simulink model "q_2dof_helicopter_quick_start"  (Simulink 8.7)
settings: Solver=ode1  StartTime=0.0  StopTime=inf  FixedStep=0.002  MaxStep=10  RelTol=1e-3  AbsTol=1e-3
libraries: sldrtlib x4, simulink_extras x4, simulink x1
settings Model: Creator=MLevis  LastModifiedBy=lukas  SimulationMode=external  ExtModeTrigDuration=50000
settings SolverCC: PositivePriorityOrder=on
settings DataIOCC: LimitDataPoints=off  SignalLoggingSaveFormat=ModelDataLogs  SaveOutput=off  SaveTime=off  SignalLoggingName=sigsOut
settings OptimizationCC: BlockReduction=off  BooleanDataType=off  OptimizeBlockIOStorage=off  BufferReuse=off  GlobalBufferReuse=off  ExpressionFolding=off  ExpressionDepthLimit=2147483647  LocalBlockOutputs=off  InitFltsAndDblsToZero=on
settings DebuggingCC: SaveWithParameterizedLinksMsg=none  SignalResolutionControl=TryResolveAllWithWarning  MultiTaskDSMMsg=warning  MultiTaskCondExecSysMsg=none  FcnCallInpInsideContextMsg=UseLocalSettings  StateNameClashWarn=warning  StrictBusMsg=None
settings RTWCC: SystemTargetFile=quarc_windows.tlc  TemplateMakefile=quarc_default_tmf  Description=QuaRC Win32 Target
settings STFCustomTargetCC: TargetFcnLib=ansi_tfl_tmw.mat  TargetPreCompLibLocation=C:\PROGRA~2\QUARC\lib\2011a\windows\release  GeneratePreprocessorConditionals=Disable all  CPPClassGenCompliant=on  SystemTargetFile=quarc_windows.tlc
settings GRTTargetCC: TargetFcnLib=ansi_tfl_tmw.mat  TargetPreCompLibLocation=C:\PROGRA~2\QUARC\lib\2011a\windows\release  ParMdlRefBuildCompliant=off  CompOptLevelCompliant=off  ConcurrentExecutionCompliant=off  CombineOutputUpdateFcns=off  MatFileLogging=off  GRTInterface=on  UseToolchainInfoCompliant=off  ExtMode=on  ExtModeMexFile=quarc_comm

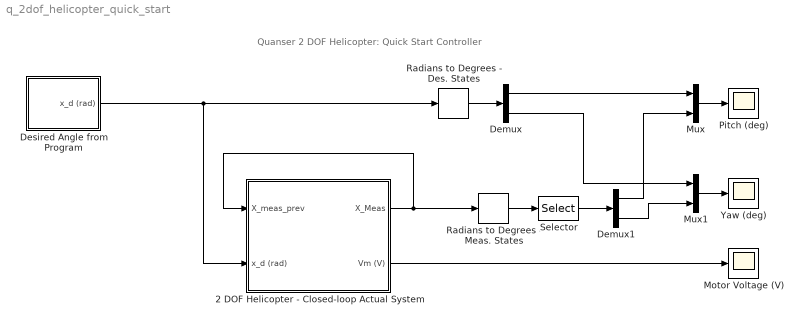
== system q_2dof_helicopter_quick_start ==
  note: Quanser 2 DOF Helicopter:
      | Quick Start Controller
  2 DOF Helicopter - Closed-loop Actual System : Subsystem
  Demux : Demux  Outputs=2
  Demux1 : Demux  Outputs=2
  Desired Angle from Program : Subsystem
  Motor Voltage (V) : Scope
  Mux : Mux  Inputs=2
  Mux1 : Mux  Inputs=2
  Pitch (deg) : Scope
  Radians to Degrees - Des. States : simulink_extras/Transformations/Radians to Degrees
  Radians to Degrees - Meas. States : simulink_extras/Transformations/Radians to Degrees
  Selector : Selector  InputPortWidth=4  IndexOptions=Index vector (dialog)  Indices=[1 2]  OutputSizes=1
  Yaw (deg) : Scope
  wires:
  2 DOF Helicopter - Closed-loop Actual System/1(X_Meas) -> 2 DOF Helicopter - Closed-loop Actual System/1(X_meas_prev), Radians to Degrees - Meas. States/1
  Desired Angle from Program/1(x_d (rad)) -> 2 DOF Helicopter - Closed-loop Actual System/2(x_d (rad)), Radians to Degrees - Des. States/1
  Radians to Degrees - Des. States/1 -> Demux/1
  Radians to Degrees - Meas. States/1 -> Selector/1
  Selector/1 -> Demux1/1
  Mux1/1 -> Yaw (deg)/1
  Mux/1 -> Pitch (deg)/1
  Demux/1 -> Mux/1
  Demux/2 -> Mux1/1
  Demux1/1 -> Mux/2
  Demux1/2 -> Mux1/2
  2 DOF Helicopter - Closed-loop Actual System/2(Vm (V)) -> Motor Voltage (V)/1

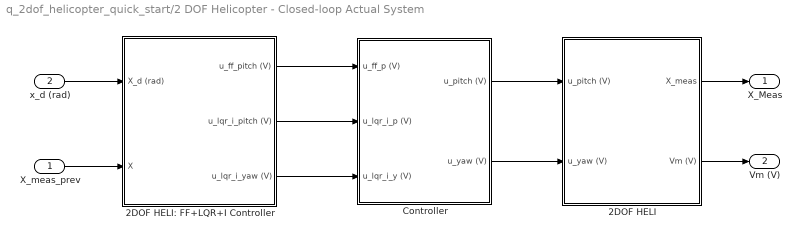
== system q_2dof_helicopter_quick_start/2 DOF Helicopter - Closed-loop Actual System ==
  X_meas_prev : Inport
  x_d (rad) : Inport  Port=2
  2DOF HELI : Subsystem
  2DOF HELI: FF+LQR+I Controller : Subsystem
  "Controller " : Subsystem
  X_Meas : Outport
  Vm (V) : Outport  Port=2
  wires:
  2DOF HELI/1(X_meas) -> X_Meas/1
  x_d (rad)/1 -> 2DOF HELI: FF+LQR+I Controller/1(X_d (rad))
  X_meas_prev/1 -> 2DOF HELI: FF+LQR+I Controller/2(X)
  "Controller "/1(u_pitch (V)) -> 2DOF HELI/1(u_pitch (V))
  "Controller "/2(u_yaw (V)) -> 2DOF HELI/2(u_yaw (V))
  2DOF HELI: FF+LQR+I Controller/2(u_lqr_i_pitch (V)) -> "Controller "/2(u_lqr_i_p (V))
  2DOF HELI: FF+LQR+I Controller/1(u_ff_pitch (V)) -> "Controller "/1(u_ff_p (V))
  2DOF HELI: FF+LQR+I Controller/3(u_lqr_i_yaw (V)) -> "Controller "/3(u_lqr_i_y (V))
  2DOF HELI/2(Vm (V)) -> Vm (V)/1

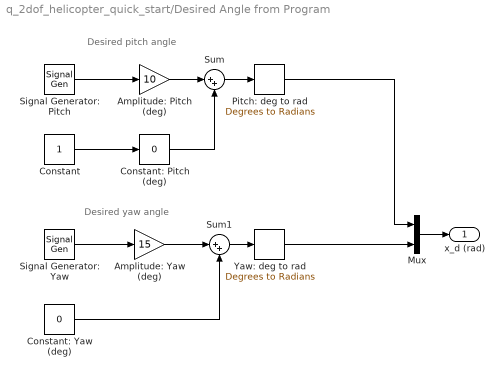
== system q_2dof_helicopter_quick_start/Desired Angle from Program ==
  note: Desired pitch angle
  note: Desired yaw angle
  Amplitude: Pitch (deg) : Gain  Gain=10
  Amplitude: Yaw (deg) : Gain  Gain=15
  Constant : Constant
  Constant: Pitch (deg) : simulink/Math Operations/Slider Gain  low=-30  gain=0  high=15
  Constant: Yaw (deg) : Constant  Value=0
  Mux : Mux  Inputs=2
  Pitch: deg to rad : simulink_extras/Transformations/Degrees to Radians
  Signal Generator: Pitch : SignalGenerator  WaveForm=square  Frequency=0.05
  Signal Generator: Yaw : SignalGenerator  WaveForm=square  Frequency=0.05
  Sum : Sum  Inputs=|++
  Sum1 : Sum  Inputs=|++
  Yaw: deg to rad : simulink_extras/Transformations/Degrees to Radians
  x_d (rad) : Outport
  wires:
  Pitch: deg to rad/1 -> Mux/1
  Sum/1 -> Pitch: deg to rad/1
  Signal Generator: Pitch/1 -> Amplitude: Pitch (deg)/1
  Amplitude: Pitch (deg)/1 -> Sum/1
  Constant/1 -> Constant: Pitch (deg)/1
  Sum1/1 -> Yaw: deg to rad/1
  Signal Generator: Yaw/1 -> Amplitude: Yaw (deg)/1
  Amplitude: Yaw (deg)/1 -> Sum1/1
  Constant: Yaw (deg)/1 -> Sum1/2
  Mux/1 -> x_d (rad)/1
  Yaw: deg to rad/1 -> Mux/2
  Constant: Pitch (deg)/1 -> Sum/2

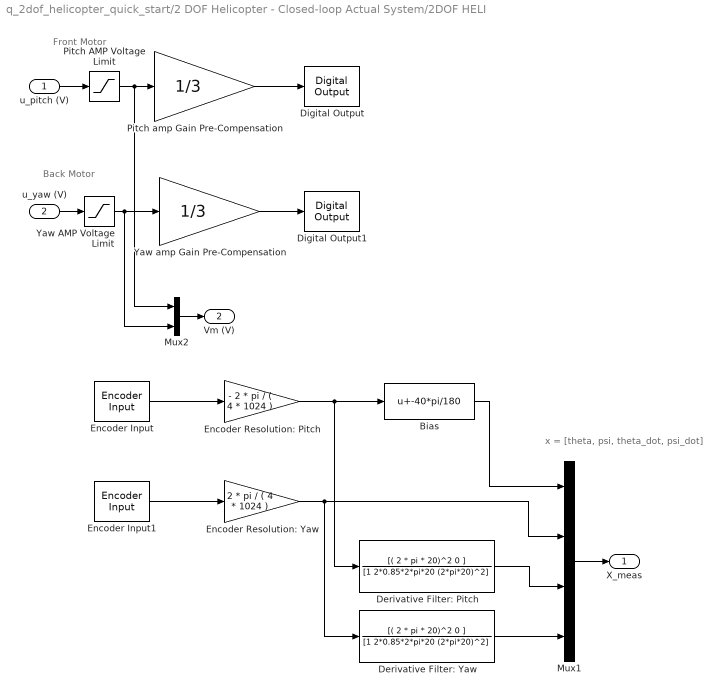
== system q_2dof_helicopter_quick_start/2 DOF Helicopter - Closed-loop Actual System/2DOF HELI ==
  note: Back Motor
  note: Front Motor
  note: x = [theta, psi, theta_dot, psi_dot]
  u_pitch (V) : Inport
  u_yaw (V) : Inport  Port=2
  Bias : Bias  Bias=-40*pi/180
  Derivative Filter: Pitch : TransferFcn  Numerator=[( 2 * pi * 20)^2 0 ]  Denominator=[1 2*0.85*2*pi*20 (2*pi*20)^2]
  Derivative Filter: Yaw : TransferFcn  Numerator=[( 2 * pi * 20)^2 0 ]  Denominator=[1 2*0.85*2*pi*20 (2*pi*20)^2]
  Digital Output : sldrtlib/Digital Output  SampleTime=0.1  MaxMissedTicks=10  ShowMissedTicks=off  YieldWhenWaiting=off  DrvAddress=0  DrvOptions=0  Channels=1  BitMode=1  InitialValue=[]  FinalValue=[]
  Digital Output1 : sldrtlib/Digital Output  SampleTime=0.1  MaxMissedTicks=10  ShowMissedTicks=off  YieldWhenWaiting=off  DrvAddress=0  DrvOptions=0  Channels=1  BitMode=1  InitialValue=[]  FinalValue=[]
  Encoder Input : sldrtlib/Encoder Input  SampleTime=0.01  MaxMissedTicks=10  ShowMissedTicks=off  YieldWhenWaiting=off  DrvAddress=0  DrvOptions=0  Channels=1  QuadMode=3  IndexPulse=2  InputFilter=Inf  DataType=1
  Encoder Input1 : sldrtlib/Encoder Input  SampleTime=0.01  MaxMissedTicks=10  ShowMissedTicks=off  YieldWhenWaiting=off  DrvAddress=0  DrvOptions=0  Channels=1  QuadMode=3  IndexPulse=2  InputFilter=Inf  DataType=1
  "Encoder Resolution: Pitch " : Gain  Gain=- 2 * pi / ( 4 * 1024 )
  Encoder Resolution: Yaw : Gain  Gain=2 * pi / ( 4 * 1024 )
  Mux1 : Mux
  Mux2 : Mux  Inputs=2
  Pitch AMP Voltage Limit : Saturate  UpperLimit=3.5  LowerLimit=-3.5
  Pitch amp Gain Pre-Compensation : Gain  Gain=1/3  SaturateOnIntegerOverflow=on  OutDataTypeStr=Inherit: Same as input  ParamDataTypeStr=Inherit: Same as input
  Yaw AMP Voltage Limit : Saturate  UpperLimit=3.5  LowerLimit=-3.5
  Yaw amp Gain Pre-Compensation : Gain  Gain=1/3  SaturateOnIntegerOverflow=on  OutDataTypeStr=Inherit: Same as input  ParamDataTypeStr=Inherit: Same as input
  X_meas : Outport
  Vm (V) : Outport  Port=2
  wires:
  Encoder Resolution: Yaw/1 -> Mux1/2, Derivative Filter: Yaw/1
  Mux2/1 -> Vm (V)/1
  Yaw amp Gain Pre-Compensation/1 -> Digital Output1/1
  Pitch amp Gain Pre-Compensation/1 -> Digital Output/1
  Mux1/1 -> X_meas/1
  u_yaw (V)/1 -> Yaw AMP Voltage Limit/1
  u_pitch (V)/1 -> Pitch AMP Voltage Limit/1
  Yaw AMP Voltage Limit/1 -> Mux2/2, Yaw amp Gain Pre-Compensation/1
  Pitch AMP Voltage Limit/1 -> Mux2/1, Pitch amp Gain Pre-Compensation/1
  Encoder Input/1 -> "Encoder Resolution: Pitch "/1
  "Encoder Resolution: Pitch "/1 -> Bias/1, Derivative Filter: Pitch/1
  Encoder Input1/1 -> Encoder Resolution: Yaw/1
  Bias/1 -> Mux1/1
  Derivative Filter: Pitch/1 -> Mux1/3
  Derivative Filter: Yaw/1 -> Mux1/4

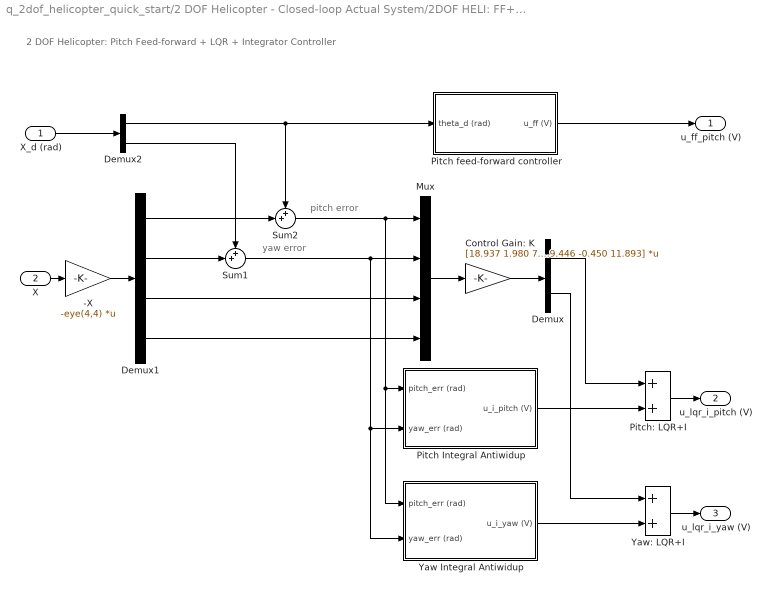
== system q_2dof_helicopter_quick_start/2 DOF Helicopter - Closed-loop Actual System/2DOF HELI: FF+LQR+I Controller ==
  note: yaw error
  note: pitch error
  note: 2 DOF Helicopter:
      | Pitch Feed-forward + LQR + Integrator Controller
  X_d (rad) : Inport
  X : Inport  Port=2
  -X : Gain  Gain=-eye(4,4)  Multiplication=Matrix(K*u)
  Control Gain: K : Gain  Gain=[18.937 1.980 7.492 1.528; -2.222 19.446 -0.450 11.893]  Multiplication=Matrix(K*u)
  Demux : Demux  Outputs=2
  Demux1 : Demux
  Demux2 : Demux  Outputs=2
  Mux : Mux
  Pitch Integral Antiwidup : Subsystem
  Pitch feed-forward controller : Subsystem
  Pitch: LQR+I : Sum
  Sum1 : Sum  Inputs=++|
  Sum2 : Sum  Inputs=++|
  Yaw Integral Antiwidup : Subsystem
  Yaw: LQR+I : Sum
  u_ff_pitch (V) : Outport
  u_lqr_i_pitch (V) : Outport  Port=2
  u_lqr_i_yaw (V) : Outport  Port=3
  wires:
  Demux1/2 -> Sum1/2
  Demux2/2 -> Sum1/1
  Demux2/1 -> Sum2/1, Pitch feed-forward controller/1(theta_d (rad))
  X_d (rad)/1 -> Demux2/1
  Yaw Integral Antiwidup/1(u_i_yaw (V)) -> Yaw: LQR+I/2
  Demux/2 -> Yaw: LQR+I/1
  Yaw: LQR+I/1 -> u_lqr_i_yaw (V)/1
  Pitch: LQR+I/1 -> u_lqr_i_pitch (V)/1
  Demux/1 -> Pitch: LQR+I/1
  Pitch Integral Antiwidup/1(u_i_pitch (V)) -> Pitch: LQR+I/2
  Pitch feed-forward controller/1(u_ff (V)) -> u_ff_pitch (V)/1
  Sum2/1 -> Mux/1, Yaw Integral Antiwidup/1(pitch_err (rad)), Pitch Integral Antiwidup/1(pitch_err (rad))
  Demux1/1 -> Sum2/2
  X/1 -> -X/1
  Sum1/1 -> Pitch Integral Antiwidup/2(yaw_err (rad)), Yaw Integral Antiwidup/2(yaw_err (rad)), Mux/2
  -X/1 -> Demux1/1
  Control Gain: K/1 -> Demux/1
  Mux/1 -> Control Gain: K/1
  Demux1/3 -> Mux/3
  Demux1/4 -> Mux/4

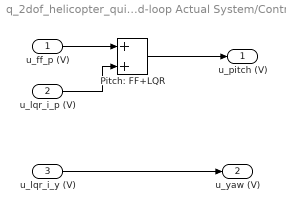
== system q_2dof_helicopter_quick_start/2 DOF Helicopter - Closed-loop Actual System/Controller  ==
  u_ff_p (V) : Inport
  u_lqr_i_p (V) : Inport  Port=2
  u_lqr_i_y (V) : Inport  Port=3
  Pitch: FF+LQR : Sum
  u_pitch (V) : Outport
  u_yaw (V) : Outport  Port=2
  wires:
  u_lqr_i_y (V)/1 -> u_yaw (V)/1
  u_lqr_i_p (V)/1 -> Pitch: FF+LQR/2
  u_ff_p (V)/1 -> Pitch: FF+LQR/1
  Pitch: FF+LQR/1 -> u_pitch (V)/1

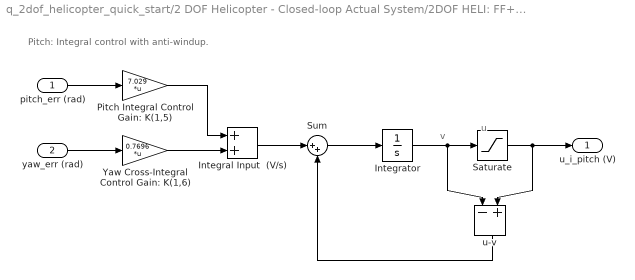
== system q_2dof_helicopter_quick_start/2 DOF Helicopter - Closed-loop Actual System/2DOF HELI: FF+LQR+I Controller/Pitch Integral Antiwidup ==
  note: Pitch: Integral control with anti-windup.
  note: v
  note: u
  pitch_err (rad) : Inport
  yaw_err (rad) : Inport  Port=2
  Integral Input  (V/s) : Sum
  Integrator : Integrator
  Pitch Integral Control Gain: K(1,5) : Gain  Gain=7.029  Multiplication=Matrix(K*u)
  Saturate : Saturate  UpperLimit=5  LowerLimit=-5
  Sum : Sum  Inputs=|++
  Yaw Cross-Integral Control Gain: K(1,6) : Gain  Gain=0.7696  Multiplication=Matrix(K*u)
  u-v : Sum  Inputs=-+
  u_i_pitch (V) : Outport
  wires:
  Integral Input  (V/s)/1 -> Sum/1
  Yaw Cross-Integral Control Gain: K(1,6)/1 -> Integral Input  (V/s)/2
  Pitch Integral Control Gain: K(1,5)/1 -> Integral Input  (V/s)/1
  yaw_err (rad)/1 -> Yaw Cross-Integral Control Gain: K(1,6)/1
  Sum/1 -> Integrator/1
  u-v/1 -> Sum/2
  Saturate/1 -> u-v/2, u_i_pitch (V)/1
  Integrator/1 -> Saturate/1, u-v/1
  pitch_err (rad)/1 -> Pitch Integral Control Gain: K(1,5)/1

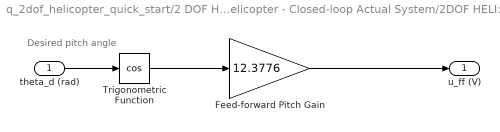
== system q_2dof_helicopter_quick_start/2 DOF Helicopter - Closed-loop Actual System/2DOF HELI: FF+LQR+I Controller/Pitch feed-forward controller ==
  note: Desired pitch angle
  theta_d (rad) : Inport
  Feed-forward Pitch Gain : Gain  Gain=12.3776
  Trigonometric Function : Trigonometry  Operator=cos  OutputSignalType=real
  u_ff (V) : Outport
  wires:
  theta_d (rad)/1 -> Trigonometric Function/1
  Feed-forward Pitch Gain/1 -> u_ff (V)/1
  Trigonometric Function/1 -> Feed-forward Pitch Gain/1

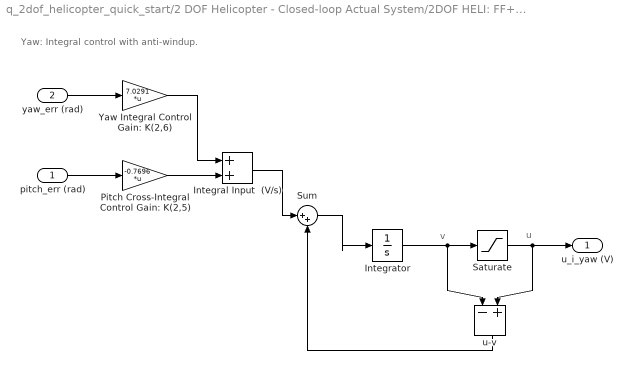
== system q_2dof_helicopter_quick_start/2 DOF Helicopter - Closed-loop Actual System/2DOF HELI: FF+LQR+I Controller/Yaw Integral Antiwidup ==
  note: Yaw: Integral control with anti-windup.
  note: u
  note: v
  pitch_err (rad) : Inport
  yaw_err (rad) : Inport  Port=2
  Integral Input  (V/s) : Sum
  Integrator : Integrator
  Pitch Cross-Integral Control Gain: K(2,5) : Gain  Gain=-0.7696  Multiplication=Matrix(K*u)
  Saturate : Saturate  UpperLimit=8  LowerLimit=-8
  Sum : Sum  Inputs=|++
  Yaw Integral Control Gain: K(2,6) : Gain  Gain=7.0291  Multiplication=Matrix(K*u)
  u-v : Sum  Inputs=-+
  u_i_yaw (V) : Outport
  wires:
  Integral Input  (V/s)/1 -> Sum/1
  Pitch Cross-Integral Control Gain: K(2,5)/1 -> Integral Input  (V/s)/2
  Yaw Integral Control Gain: K(2,6)/1 -> Integral Input  (V/s)/1
  pitch_err (rad)/1 -> Pitch Cross-Integral Control Gain: K(2,5)/1
  yaw_err (rad)/1 -> Yaw Integral Control Gain: K(2,6)/1
  Integrator/1 -> u-v/1, Saturate/1
  Saturate/1 -> u_i_yaw (V)/1, u-v/2
  u-v/1 -> Sum/2
  Sum/1 -> Integrator/1
